simulink model "WindFarm_2023_BaseModel_v2"  (R2019a)
settings: Solver=ode1  StartTime=0.0  StopTime=2  FixedStep=Ts_Power  RelTol=1e-3
PostLoadFcn:
  | %% Init for wind PnO models - global system parameters
  | OVERRIDE_SSN_MEMORY_LIMIT=1;
  | Ts=50e-6;
  | % Ts=50e-10;
  | Ts_Power=Ts;
  | Ts_Control=2*Ts;
  | freq = 50;
  | Fnom=freq;
  | Vac=400e3;
InitFcn:
  | %% Init for wind PnO models - global system parameters
  | OVERRIDE_SSN_MEMORY_LIMIT=1;
  | Ts=50e-6;
  | % Ts=50e-10;
  | Ts_Power=Ts;
  | Ts_Control=2*Ts;
  | freq = 50;
  | Fnom=freq;
  | Vac=400e3;
undefined symbols (not defined in the file or in its folder): Bessel, Butterworth, Complex, D11, Delta, den, DiscIntNeverNeededParam, dx, find_system, gcbh, Iabc, No, num, out_Buses, out_WindFarms, sps_rtmsupport, Vabc, WindFarm_Selection_1, yes
libraries: powerlib x1158, simulink x592, powerlib_meascontrol x592, eeSinusoidalMeasurement x212, simulink_extras x104, elements x52, eePowerMeasurement x50, spsVIMeasurementModel x45
(part 82 of 86)

== system WindFarm_2023_BaseModel_v2/SM_WT1/Wind Type IV Detailed v2.1 - 2/Control/Measurement and Transformation/Discrete 3-phase PLL-Driven Positive-Sequence Active & Reactive Power/Discrete 3-phase PLL-Driven Positive-Sequence Fundamental Value2/Discrete Variable Frequency Mean value1/Correction subsystem ==
  N : Inport
  F : Inport  Port=2
  In : Inport  Port=3
  Gain1 : Gain  Gain=0.5  SaturateOnIntegerOverflow=on  OutDataTypeStr=Inherit: Same as input  ParamDataTypeStr=Inherit: Same as input
  Product2 : Product  Inputs=*/  SaturateOnIntegerOverflow=on  InputSameDT=on  OutDataTypeStr=Inherit: Same as first input
  Product4 : Product  Inputs=**  SaturateOnIntegerOverflow=on  InputSameDT=on  OutDataTypeStr=Inherit: Same as first input
  Product5 : Product  Inputs=**  SaturateOnIntegerOverflow=on  InputSameDT=on  OutDataTypeStr=Inherit: Same as first input
  Sum1 : Sum  Inputs=+-  SaturateOnIntegerOverflow=on  InputSameDT=on  OutDataTypeStr=Inherit: Same as first input
  Sum4 : Sum  SaturateOnIntegerOverflow=on  InputSameDT=on  OutDataTypeStr=Inherit: Same as first input
  Sum5 : Sum  Inputs=+-  SaturateOnIntegerOverflow=on  InputSameDT=on  OutDataTypeStr=Inherit: Same as first input
  Unit Delay : UnitDelay  SampleTime=Ts  HasFrameUpgradeWarning=on
  Out : Outport  VectorParamsAs1DForOutWhenUnconnected=on
  wires:
  Product4/1 -> Out/1
  Sum4/1 -> Product4/2
  Gain1/1 -> Sum4/1
  Product5/1 -> Gain1/1
  Sum1/1 -> Product5/2
  In/1 -> Sum4/2, Unit Delay/1, Sum1/1
  Product2/1 -> Product4/1
  Sum5/1 -> Product5/1, Product2/1
  F/1 -> Sum5/2
  N/1 -> Product2/2, Sum5/1
  Unit Delay/1 -> Sum1/2

== system WindFarm_2023_BaseModel_v2/SM_WT1/Wind Type IV Detailed v2.1 - 2/Control/Measurement and Transformation/Discrete 3-phase PLL-Driven Positive-Sequence Active & Reactive Power/Discrete 3-phase PLL-Driven Positive-Sequence Fundamental Value2/Discrete Variable Frequency Mean value1/Discrete Variable Transport Delay ==
  In : Inport
  D : Inport  Port=2
  "S-Function " : S-Function  FunctionName=discreteVariableTransportDelay  Parameters=MaxDelay,Ts,InitialValue  SFunctionDeploymentMode=off  EnableBusSupport=off
  Out : Outport  VectorParamsAs1DForOutWhenUnconnected=on
  wires:
  D/1 -> "S-Function "/2
  In/1 -> "S-Function "/1
  "S-Function "/1 -> Out/1

== system WindFarm_2023_BaseModel_v2/SM_WT1/Wind Type IV Detailed v2.1 - 2/Control/Measurement and Transformation/Discrete 3-phase PLL-Driven Positive-Sequence Active & Reactive Power/Discrete 3-phase PLL-Driven Positive-Sequence Fundamental Value2/Discrete Variable Frequency Mean value2/Correction subsystem ==
  N : Inport
  F : Inport  Port=2
  In : Inport  Port=3
  Gain1 : Gain  Gain=0.5  SaturateOnIntegerOverflow=on  OutDataTypeStr=Inherit: Same as input  ParamDataTypeStr=Inherit: Same as input
  Product2 : Product  Inputs=*/  SaturateOnIntegerOverflow=on  InputSameDT=on  OutDataTypeStr=Inherit: Same as first input
  Product4 : Product  Inputs=**  SaturateOnIntegerOverflow=on  InputSameDT=on  OutDataTypeStr=Inherit: Same as first input
  Product5 : Product  Inputs=**  SaturateOnIntegerOverflow=on  InputSameDT=on  OutDataTypeStr=Inherit: Same as first input
  Sum1 : Sum  Inputs=+-  SaturateOnIntegerOverflow=on  InputSameDT=on  OutDataTypeStr=Inherit: Same as first input
  Sum4 : Sum  SaturateOnIntegerOverflow=on  InputSameDT=on  OutDataTypeStr=Inherit: Same as first input
  Sum5 : Sum  Inputs=+-  SaturateOnIntegerOverflow=on  InputSameDT=on  OutDataTypeStr=Inherit: Same as first input
  Unit Delay : UnitDelay  SampleTime=Ts  HasFrameUpgradeWarning=on
  Out : Outport  VectorParamsAs1DForOutWhenUnconnected=on
  wires:
  Unit Delay/1 -> Sum1/2
  N/1 -> Sum5/1, Product2/2
  F/1 -> Sum5/2
  Sum5/1 -> Product2/1, Product5/1
  Product2/1 -> Product4/1
  In/1 -> Sum1/1, Unit Delay/1, Sum4/2
  Sum1/1 -> Product5/2
  Product5/1 -> Gain1/1
  Gain1/1 -> Sum4/1
  Sum4/1 -> Product4/2
  Product4/1 -> Out/1

== system WindFarm_2023_BaseModel_v2/SM_WT1/Wind Type IV Detailed v2.1 - 2/Control/Measurement and Transformation/Discrete 3-phase PLL-Driven Positive-Sequence Active & Reactive Power/Discrete 3-phase PLL-Driven Positive-Sequence Fundamental Value2/Discrete Variable Frequency Mean value2/Discrete Variable Transport Delay ==
  In : Inport
  D : Inport  Port=2
  "S-Function " : S-Function  FunctionName=discreteVariableTransportDelay  Parameters=MaxDelay,Ts,InitialValue  SFunctionDeploymentMode=off  EnableBusSupport=off
  Out : Outport  VectorParamsAs1DForOutWhenUnconnected=on
  wires:
  "S-Function "/1 -> Out/1
  In/1 -> "S-Function "/1
  D/1 -> "S-Function "/2

== system WindFarm_2023_BaseModel_v2/SM_WT1/Wind Type IV Detailed v2.1 - 20/Control/Measurement and Transformation/Discrete 3-phase PLL-Driven Positive-Sequence Active & Reactive Power/Discrete 3-phase PLL-Driven Positive-Sequence Fundamental Value/Discrete Variable Frequency Mean value1/Correction subsystem ==
  N : Inport
  F : Inport  Port=2
  In : Inport  Port=3
  Gain1 : Gain  Gain=0.5  SaturateOnIntegerOverflow=on  OutDataTypeStr=Inherit: Same as input  ParamDataTypeStr=Inherit: Same as input
  Product2 : Product  Inputs=*/  SaturateOnIntegerOverflow=on  InputSameDT=on  OutDataTypeStr=Inherit: Same as first input
  Product4 : Product  Inputs=**  SaturateOnIntegerOverflow=on  InputSameDT=on  OutDataTypeStr=Inherit: Same as first input
  Product5 : Product  Inputs=**  SaturateOnIntegerOverflow=on  InputSameDT=on  OutDataTypeStr=Inherit: Same as first input
  Sum1 : Sum  Inputs=+-  SaturateOnIntegerOverflow=on  InputSameDT=on  OutDataTypeStr=Inherit: Same as first input
  Sum4 : Sum  SaturateOnIntegerOverflow=on  InputSameDT=on  OutDataTypeStr=Inherit: Same as first input
  Sum5 : Sum  Inputs=+-  SaturateOnIntegerOverflow=on  InputSameDT=on  OutDataTypeStr=Inherit: Same as first input
  Unit Delay : UnitDelay  SampleTime=Ts  HasFrameUpgradeWarning=on
  Out : Outport  VectorParamsAs1DForOutWhenUnconnected=on
  wires:
  Product4/1 -> Out/1
  Sum4/1 -> Product4/2
  Gain1/1 -> Sum4/1
  Product5/1 -> Gain1/1
  Sum1/1 -> Product5/2
  In/1 -> Sum4/2, Unit Delay/1, Sum1/1
  Product2/1 -> Product4/1
  Sum5/1 -> Product5/1, Product2/1
  F/1 -> Sum5/2
  N/1 -> Product2/2, Sum5/1
  Unit Delay/1 -> Sum1/2

== system WindFarm_2023_BaseModel_v2/SM_WT1/Wind Type IV Detailed v2.1 - 20/Control/Measurement and Transformation/Discrete 3-phase PLL-Driven Positive-Sequence Active & Reactive Power/Discrete 3-phase PLL-Driven Positive-Sequence Fundamental Value/Discrete Variable Frequency Mean value1/Discrete Variable Transport Delay ==
  In : Inport
  D : Inport  Port=2
  "S-Function " : S-Function  FunctionName=discreteVariableTransportDelay  Parameters=MaxDelay,Ts,InitialValue  SFunctionDeploymentMode=off  EnableBusSupport=off
  Out : Outport  VectorParamsAs1DForOutWhenUnconnected=on
  wires:
  D/1 -> "S-Function "/2
  In/1 -> "S-Function "/1
  "S-Function "/1 -> Out/1

== system WindFarm_2023_BaseModel_v2/SM_WT1/Wind Type IV Detailed v2.1 - 20/Control/Measurement and Transformation/Discrete 3-phase PLL-Driven Positive-Sequence Active & Reactive Power/Discrete 3-phase PLL-Driven Positive-Sequence Fundamental Value/Discrete Variable Frequency Mean value2/Correction subsystem ==
  N : Inport
  F : Inport  Port=2
  In : Inport  Port=3
  Gain1 : Gain  Gain=0.5  SaturateOnIntegerOverflow=on  OutDataTypeStr=Inherit: Same as input  ParamDataTypeStr=Inherit: Same as input
  Product2 : Product  Inputs=*/  SaturateOnIntegerOverflow=on  InputSameDT=on  OutDataTypeStr=Inherit: Same as first input
  Product4 : Product  Inputs=**  SaturateOnIntegerOverflow=on  InputSameDT=on  OutDataTypeStr=Inherit: Same as first input
  Product5 : Product  Inputs=**  SaturateOnIntegerOverflow=on  InputSameDT=on  OutDataTypeStr=Inherit: Same as first input
  Sum1 : Sum  Inputs=+-  SaturateOnIntegerOverflow=on  InputSameDT=on  OutDataTypeStr=Inherit: Same as first input
  Sum4 : Sum  SaturateOnIntegerOverflow=on  InputSameDT=on  OutDataTypeStr=Inherit: Same as first input
  Sum5 : Sum  Inputs=+-  SaturateOnIntegerOverflow=on  InputSameDT=on  OutDataTypeStr=Inherit: Same as first input
  Unit Delay : UnitDelay  SampleTime=Ts  HasFrameUpgradeWarning=on
  Out : Outport  VectorParamsAs1DForOutWhenUnconnected=on
  wires:
  Unit Delay/1 -> Sum1/2
  N/1 -> Sum5/1, Product2/2
  F/1 -> Sum5/2
  Sum5/1 -> Product2/1, Product5/1
  Product2/1 -> Product4/1
  In/1 -> Sum1/1, Unit Delay/1, Sum4/2
  Sum1/1 -> Product5/2
  Product5/1 -> Gain1/1
  Gain1/1 -> Sum4/1
  Sum4/1 -> Product4/2
  Product4/1 -> Out/1

== system WindFarm_2023_BaseModel_v2/SM_WT1/Wind Type IV Detailed v2.1 - 20/Control/Measurement and Transformation/Discrete 3-phase PLL-Driven Positive-Sequence Active & Reactive Power/Discrete 3-phase PLL-Driven Positive-Sequence Fundamental Value/Discrete Variable Frequency Mean value2/Discrete Variable Transport Delay ==
  In : Inport
  D : Inport  Port=2
  "S-Function " : S-Function  FunctionName=discreteVariableTransportDelay  Parameters=MaxDelay,Ts,InitialValue  SFunctionDeploymentMode=off  EnableBusSupport=off
  Out : Outport  VectorParamsAs1DForOutWhenUnconnected=on
  wires:
  "S-Function "/1 -> Out/1
  In/1 -> "S-Function "/1
  D/1 -> "S-Function "/2

== system WindFarm_2023_BaseModel_v2/SM_WT1/Wind Type IV Detailed v2.1 - 20/Control/Measurement and Transformation/Discrete 3-phase PLL-Driven Positive-Sequence Active & Reactive Power/Discrete 3-phase PLL-Driven Positive-Sequence Fundamental Value2/Discrete Variable Frequency Mean value1/Correction subsystem ==
  N : Inport
  F : Inport  Port=2
  In : Inport  Port=3
  Gain1 : Gain  Gain=0.5  SaturateOnIntegerOverflow=on  OutDataTypeStr=Inherit: Same as input  ParamDataTypeStr=Inherit: Same as input
  Product2 : Product  Inputs=*/  SaturateOnIntegerOverflow=on  InputSameDT=on  OutDataTypeStr=Inherit: Same as first input
  Product4 : Product  Inputs=**  SaturateOnIntegerOverflow=on  InputSameDT=on  OutDataTypeStr=Inherit: Same as first input
  Product5 : Product  Inputs=**  SaturateOnIntegerOverflow=on  InputSameDT=on  OutDataTypeStr=Inherit: Same as first input
  Sum1 : Sum  Inputs=+-  SaturateOnIntegerOverflow=on  InputSameDT=on  OutDataTypeStr=Inherit: Same as first input
  Sum4 : Sum  SaturateOnIntegerOverflow=on  InputSameDT=on  OutDataTypeStr=Inherit: Same as first input
  Sum5 : Sum  Inputs=+-  SaturateOnIntegerOverflow=on  InputSameDT=on  OutDataTypeStr=Inherit: Same as first input
  Unit Delay : UnitDelay  SampleTime=Ts  HasFrameUpgradeWarning=on
  Out : Outport  VectorParamsAs1DForOutWhenUnconnected=on
  wires:
  Unit Delay/1 -> Sum1/2
  N/1 -> Sum5/1, Product2/2
  F/1 -> Sum5/2
  Sum5/1 -> Product2/1, Product5/1
  Product2/1 -> Product4/1
  In/1 -> Sum1/1, Unit Delay/1, Sum4/2
  Sum1/1 -> Product5/2
  Product5/1 -> Gain1/1
  Gain1/1 -> Sum4/1
  Sum4/1 -> Product4/2
  Product4/1 -> Out/1

== system WindFarm_2023_BaseModel_v2/SM_WT1/Wind Type IV Detailed v2.1 - 20/Control/Measurement and Transformation/Discrete 3-phase PLL-Driven Positive-Sequence Active & Reactive Power/Discrete 3-phase PLL-Driven Positive-Sequence Fundamental Value2/Discrete Variable Frequency Mean value1/Discrete Variable Transport Delay ==
  In : Inport
  D : Inport  Port=2
  "S-Function " : S-Function  FunctionName=discreteVariableTransportDelay  Parameters=MaxDelay,Ts,InitialValue  SFunctionDeploymentMode=off  EnableBusSupport=off
  Out : Outport  VectorParamsAs1DForOutWhenUnconnected=on
  wires:
  "S-Function "/1 -> Out/1
  In/1 -> "S-Function "/1
  D/1 -> "S-Function "/2

== system WindFarm_2023_BaseModel_v2/SM_WT1/Wind Type IV Detailed v2.1 - 20/Control/Measurement and Transformation/Discrete 3-phase PLL-Driven Positive-Sequence Active & Reactive Power/Discrete 3-phase PLL-Driven Positive-Sequence Fundamental Value2/Discrete Variable Frequency Mean value2/Correction subsystem ==
  N : Inport
  F : Inport  Port=2
  In : Inport  Port=3
  Gain1 : Gain  Gain=0.5  SaturateOnIntegerOverflow=on  OutDataTypeStr=Inherit: Same as input  ParamDataTypeStr=Inherit: Same as input
  Product2 : Product  Inputs=*/  SaturateOnIntegerOverflow=on  InputSameDT=on  OutDataTypeStr=Inherit: Same as first input
  Product4 : Product  Inputs=**  SaturateOnIntegerOverflow=on  InputSameDT=on  OutDataTypeStr=Inherit: Same as first input
  Product5 : Product  Inputs=**  SaturateOnIntegerOverflow=on  InputSameDT=on  OutDataTypeStr=Inherit: Same as first input
  Sum1 : Sum  Inputs=+-  SaturateOnIntegerOverflow=on  InputSameDT=on  OutDataTypeStr=Inherit: Same as first input
  Sum4 : Sum  SaturateOnIntegerOverflow=on  InputSameDT=on  OutDataTypeStr=Inherit: Same as first input
  Sum5 : Sum  Inputs=+-  SaturateOnIntegerOverflow=on  InputSameDT=on  OutDataTypeStr=Inherit: Same as first input
  Unit Delay : UnitDelay  SampleTime=Ts  HasFrameUpgradeWarning=on
  Out : Outport  VectorParamsAs1DForOutWhenUnconnected=on
  wires:
  Product4/1 -> Out/1
  Sum4/1 -> Product4/2
  Gain1/1 -> Sum4/1
  Product5/1 -> Gain1/1
  Sum1/1 -> Product5/2
  In/1 -> Sum4/2, Unit Delay/1, Sum1/1
  Product2/1 -> Product4/1
  Sum5/1 -> Product5/1, Product2/1
  F/1 -> Sum5/2
  N/1 -> Product2/2, Sum5/1
  Unit Delay/1 -> Sum1/2

== system WindFarm_2023_BaseModel_v2/SM_WT1/Wind Type IV Detailed v2.1 - 20/Control/Measurement and Transformation/Discrete 3-phase PLL-Driven Positive-Sequence Active & Reactive Power/Discrete 3-phase PLL-Driven Positive-Sequence Fundamental Value2/Discrete Variable Frequency Mean value2/Discrete Variable Transport Delay ==
  In : Inport
  D : Inport  Port=2
  "S-Function " : S-Function  FunctionName=discreteVariableTransportDelay  Parameters=MaxDelay,Ts,InitialValue  SFunctionDeploymentMode=off  EnableBusSupport=off
  Out : Outport  VectorParamsAs1DForOutWhenUnconnected=on
  wires:
  D/1 -> "S-Function "/2
  In/1 -> "S-Function "/1
  "S-Function "/1 -> Out/1

== system WindFarm_2023_BaseModel_v2/SM_WT1/Wind Type IV Detailed v2.1 - 21/Control/Measurement and Transformation/Discrete 3-phase PLL-Driven Positive-Sequence Active & Reactive Power/Discrete 3-phase PLL-Driven Positive-Sequence Fundamental Value/Discrete Variable Frequency Mean value1/Correction subsystem ==
  N : Inport
  F : Inport  Port=2
  In : Inport  Port=3
  Gain1 : Gain  Gain=0.5  SaturateOnIntegerOverflow=on  OutDataTypeStr=Inherit: Same as input  ParamDataTypeStr=Inherit: Same as input
  Product2 : Product  Inputs=*/  SaturateOnIntegerOverflow=on  InputSameDT=on  OutDataTypeStr=Inherit: Same as first input
  Product4 : Product  Inputs=**  SaturateOnIntegerOverflow=on  InputSameDT=on  OutDataTypeStr=Inherit: Same as first input
  Product5 : Product  Inputs=**  SaturateOnIntegerOverflow=on  InputSameDT=on  OutDataTypeStr=Inherit: Same as first input
  Sum1 : Sum  Inputs=+-  SaturateOnIntegerOverflow=on  InputSameDT=on  OutDataTypeStr=Inherit: Same as first input
  Sum4 : Sum  SaturateOnIntegerOverflow=on  InputSameDT=on  OutDataTypeStr=Inherit: Same as first input
  Sum5 : Sum  Inputs=+-  SaturateOnIntegerOverflow=on  InputSameDT=on  OutDataTypeStr=Inherit: Same as first input
  Unit Delay : UnitDelay  SampleTime=Ts  HasFrameUpgradeWarning=on
  Out : Outport  VectorParamsAs1DForOutWhenUnconnected=on
  wires:
  Product4/1 -> Out/1
  Sum4/1 -> Product4/2
  Gain1/1 -> Sum4/1
  Product5/1 -> Gain1/1
  Sum1/1 -> Product5/2
  In/1 -> Sum4/2, Unit Delay/1, Sum1/1
  Product2/1 -> Product4/1
  Sum5/1 -> Product5/1, Product2/1
  F/1 -> Sum5/2
  N/1 -> Product2/2, Sum5/1
  Unit Delay/1 -> Sum1/2

== system WindFarm_2023_BaseModel_v2/SM_WT1/Wind Type IV Detailed v2.1 - 21/Control/Measurement and Transformation/Discrete 3-phase PLL-Driven Positive-Sequence Active & Reactive Power/Discrete 3-phase PLL-Driven Positive-Sequence Fundamental Value/Discrete Variable Frequency Mean value1/Discrete Variable Transport Delay ==
  In : Inport
  D : Inport  Port=2
  "S-Function " : S-Function  FunctionName=discreteVariableTransportDelay  Parameters=MaxDelay,Ts,InitialValue  SFunctionDeploymentMode=off  EnableBusSupport=off
  Out : Outport  VectorParamsAs1DForOutWhenUnconnected=on
  wires:
  D/1 -> "S-Function "/2
  In/1 -> "S-Function "/1
  "S-Function "/1 -> Out/1

== system WindFarm_2023_BaseModel_v2/SM_WT1/Wind Type IV Detailed v2.1 - 21/Control/Measurement and Transformation/Discrete 3-phase PLL-Driven Positive-Sequence Active & Reactive Power/Discrete 3-phase PLL-Driven Positive-Sequence Fundamental Value/Discrete Variable Frequency Mean value2/Correction subsystem ==
  N : Inport
  F : Inport  Port=2
  In : Inport  Port=3
  Gain1 : Gain  Gain=0.5  SaturateOnIntegerOverflow=on  OutDataTypeStr=Inherit: Same as input  ParamDataTypeStr=Inherit: Same as input
  Product2 : Product  Inputs=*/  SaturateOnIntegerOverflow=on  InputSameDT=on  OutDataTypeStr=Inherit: Same as first input
  Product4 : Product  Inputs=**  SaturateOnIntegerOverflow=on  InputSameDT=on  OutDataTypeStr=Inherit: Same as first input
  Product5 : Product  Inputs=**  SaturateOnIntegerOverflow=on  InputSameDT=on  OutDataTypeStr=Inherit: Same as first input
  Sum1 : Sum  Inputs=+-  SaturateOnIntegerOverflow=on  InputSameDT=on  OutDataTypeStr=Inherit: Same as first input
  Sum4 : Sum  SaturateOnIntegerOverflow=on  InputSameDT=on  OutDataTypeStr=Inherit: Same as first input
  Sum5 : Sum  Inputs=+-  SaturateOnIntegerOverflow=on  InputSameDT=on  OutDataTypeStr=Inherit: Same as first input
  Unit Delay : UnitDelay  SampleTime=Ts  HasFrameUpgradeWarning=on
  Out : Outport  VectorParamsAs1DForOutWhenUnconnected=on
  wires:
  Unit Delay/1 -> Sum1/2
  N/1 -> Sum5/1, Product2/2
  F/1 -> Sum5/2
  Sum5/1 -> Product2/1, Product5/1
  Product2/1 -> Product4/1
  In/1 -> Sum1/1, Unit Delay/1, Sum4/2
  Sum1/1 -> Product5/2
  Product5/1 -> Gain1/1
  Gain1/1 -> Sum4/1
  Sum4/1 -> Product4/2
  Product4/1 -> Out/1

== system WindFarm_2023_BaseModel_v2/SM_WT1/Wind Type IV Detailed v2.1 - 21/Control/Measurement and Transformation/Discrete 3-phase PLL-Driven Positive-Sequence Active & Reactive Power/Discrete 3-phase PLL-Driven Positive-Sequence Fundamental Value/Discrete Variable Frequency Mean value2/Discrete Variable Transport Delay ==
  In : Inport
  D : Inport  Port=2
  "S-Function " : S-Function  FunctionName=discreteVariableTransportDelay  Parameters=MaxDelay,Ts,InitialValue  SFunctionDeploymentMode=off  EnableBusSupport=off
  Out : Outport  VectorParamsAs1DForOutWhenUnconnected=on
  wires:
  "S-Function "/1 -> Out/1
  In/1 -> "S-Function "/1
  D/1 -> "S-Function "/2

== system WindFarm_2023_BaseModel_v2/SM_WT1/Wind Type IV Detailed v2.1 - 21/Control/Measurement and Transformation/Discrete 3-phase PLL-Driven Positive-Sequence Active & Reactive Power/Discrete 3-phase PLL-Driven Positive-Sequence Fundamental Value2/Discrete Variable Frequency Mean value1/Correction subsystem ==
  N : Inport
  F : Inport  Port=2
  In : Inport  Port=3
  Gain1 : Gain  Gain=0.5  SaturateOnIntegerOverflow=on  OutDataTypeStr=Inherit: Same as input  ParamDataTypeStr=Inherit: Same as input
  Product2 : Product  Inputs=*/  SaturateOnIntegerOverflow=on  InputSameDT=on  OutDataTypeStr=Inherit: Same as first input
  Product4 : Product  Inputs=**  SaturateOnIntegerOverflow=on  InputSameDT=on  OutDataTypeStr=Inherit: Same as first input
  Product5 : Product  Inputs=**  SaturateOnIntegerOverflow=on  InputSameDT=on  OutDataTypeStr=Inherit: Same as first input
  Sum1 : Sum  Inputs=+-  SaturateOnIntegerOverflow=on  InputSameDT=on  OutDataTypeStr=Inherit: Same as first input
  Sum4 : Sum  SaturateOnIntegerOverflow=on  InputSameDT=on  OutDataTypeStr=Inherit: Same as first input
  Sum5 : Sum  Inputs=+-  SaturateOnIntegerOverflow=on  InputSameDT=on  OutDataTypeStr=Inherit: Same as first input
  Unit Delay : UnitDelay  SampleTime=Ts  HasFrameUpgradeWarning=on
  Out : Outport  VectorParamsAs1DForOutWhenUnconnected=on
  wires:
  Unit Delay/1 -> Sum1/2
  N/1 -> Sum5/1, Product2/2
  F/1 -> Sum5/2
  Sum5/1 -> Product2/1, Product5/1
  Product2/1 -> Product4/1
  In/1 -> Sum1/1, Unit Delay/1, Sum4/2
  Sum1/1 -> Product5/2
  Product5/1 -> Gain1/1
  Gain1/1 -> Sum4/1
  Sum4/1 -> Product4/2
  Product4/1 -> Out/1

== system WindFarm_2023_BaseModel_v2/SM_WT1/Wind Type IV Detailed v2.1 - 21/Control/Measurement and Transformation/Discrete 3-phase PLL-Driven Positive-Sequence Active & Reactive Power/Discrete 3-phase PLL-Driven Positive-Sequence Fundamental Value2/Discrete Variable Frequency Mean value1/Discrete Variable Transport Delay ==
  In : Inport
  D : Inport  Port=2
  "S-Function " : S-Function  FunctionName=discreteVariableTransportDelay  Parameters=MaxDelay,Ts,InitialValue  SFunctionDeploymentMode=off  EnableBusSupport=off
  Out : Outport  VectorParamsAs1DForOutWhenUnconnected=on
  wires:
  "S-Function "/1 -> Out/1
  In/1 -> "S-Function "/1
  D/1 -> "S-Function "/2

== system WindFarm_2023_BaseModel_v2/SM_WT1/Wind Type IV Detailed v2.1 - 21/Control/Measurement and Transformation/Discrete 3-phase PLL-Driven Positive-Sequence Active & Reactive Power/Discrete 3-phase PLL-Driven Positive-Sequence Fundamental Value2/Discrete Variable Frequency Mean value2/Correction subsystem ==
  N : Inport
  F : Inport  Port=2
  In : Inport  Port=3
  Gain1 : Gain  Gain=0.5  SaturateOnIntegerOverflow=on  OutDataTypeStr=Inherit: Same as input  ParamDataTypeStr=Inherit: Same as input
  Product2 : Product  Inputs=*/  SaturateOnIntegerOverflow=on  InputSameDT=on  OutDataTypeStr=Inherit: Same as first input
  Product4 : Product  Inputs=**  SaturateOnIntegerOverflow=on  InputSameDT=on  OutDataTypeStr=Inherit: Same as first input
  Product5 : Product  Inputs=**  SaturateOnIntegerOverflow=on  InputSameDT=on  OutDataTypeStr=Inherit: Same as first input
  Sum1 : Sum  Inputs=+-  SaturateOnIntegerOverflow=on  InputSameDT=on  OutDataTypeStr=Inherit: Same as first input
  Sum4 : Sum  SaturateOnIntegerOverflow=on  InputSameDT=on  OutDataTypeStr=Inherit: Same as first input
  Sum5 : Sum  Inputs=+-  SaturateOnIntegerOverflow=on  InputSameDT=on  OutDataTypeStr=Inherit: Same as first input
  Unit Delay : UnitDelay  SampleTime=Ts  HasFrameUpgradeWarning=on
  Out : Outport  VectorParamsAs1DForOutWhenUnconnected=on
  wires:
  Product4/1 -> Out/1
  Sum4/1 -> Product4/2
  Gain1/1 -> Sum4/1
  Product5/1 -> Gain1/1
  Sum1/1 -> Product5/2
  In/1 -> Sum4/2, Unit Delay/1, Sum1/1
  Product2/1 -> Product4/1
  Sum5/1 -> Product5/1, Product2/1
  F/1 -> Sum5/2
  N/1 -> Product2/2, Sum5/1
  Unit Delay/1 -> Sum1/2

== system WindFarm_2023_BaseModel_v2/SM_WT1/Wind Type IV Detailed v2.1 - 21/Control/Measurement and Transformation/Discrete 3-phase PLL-Driven Positive-Sequence Active & Reactive Power/Discrete 3-phase PLL-Driven Positive-Sequence Fundamental Value2/Discrete Variable Frequency Mean value2/Discrete Variable Transport Delay ==
  In : Inport
  D : Inport  Port=2
  "S-Function " : S-Function  FunctionName=discreteVariableTransportDelay  Parameters=MaxDelay,Ts,InitialValue  SFunctionDeploymentMode=off  EnableBusSupport=off
  Out : Outport  VectorParamsAs1DForOutWhenUnconnected=on
  wires:
  D/1 -> "S-Function "/2
  In/1 -> "S-Function "/1
  "S-Function "/1 -> Out/1

== system WindFarm_2023_BaseModel_v2/SM_WT1/Wind Type IV Detailed v2.1 - 22/Control/Measurement and Transformation/Discrete 3-phase PLL-Driven Positive-Sequence Active & Reactive Power/Discrete 3-phase PLL-Driven Positive-Sequence Fundamental Value/Discrete Variable Frequency Mean value1/Correction subsystem ==
  N : Inport
  F : Inport  Port=2
  In : Inport  Port=3
  Gain1 : Gain  Gain=0.5  SaturateOnIntegerOverflow=on  OutDataTypeStr=Inherit: Same as input  ParamDataTypeStr=Inherit: Same as input
  Product2 : Product  Inputs=*/  SaturateOnIntegerOverflow=on  InputSameDT=on  OutDataTypeStr=Inherit: Same as first input
  Product4 : Product  Inputs=**  SaturateOnIntegerOverflow=on  InputSameDT=on  OutDataTypeStr=Inherit: Same as first input
  Product5 : Product  Inputs=**  SaturateOnIntegerOverflow=on  InputSameDT=on  OutDataTypeStr=Inherit: Same as first input
  Sum1 : Sum  Inputs=+-  SaturateOnIntegerOverflow=on  InputSameDT=on  OutDataTypeStr=Inherit: Same as first input
  Sum4 : Sum  SaturateOnIntegerOverflow=on  InputSameDT=on  OutDataTypeStr=Inherit: Same as first input
  Sum5 : Sum  Inputs=+-  SaturateOnIntegerOverflow=on  InputSameDT=on  OutDataTypeStr=Inherit: Same as first input
  Unit Delay : UnitDelay  SampleTime=Ts  HasFrameUpgradeWarning=on
  Out : Outport  VectorParamsAs1DForOutWhenUnconnected=on
  wires:
  Product4/1 -> Out/1
  Sum4/1 -> Product4/2
  Gain1/1 -> Sum4/1
  Product5/1 -> Gain1/1
  Sum1/1 -> Product5/2
  In/1 -> Sum4/2, Unit Delay/1, Sum1/1
  Product2/1 -> Product4/1
  Sum5/1 -> Product5/1, Product2/1
  F/1 -> Sum5/2
  N/1 -> Product2/2, Sum5/1
  Unit Delay/1 -> Sum1/2

== system WindFarm_2023_BaseModel_v2/SM_WT1/Wind Type IV Detailed v2.1 - 22/Control/Measurement and Transformation/Discrete 3-phase PLL-Driven Positive-Sequence Active & Reactive Power/Discrete 3-phase PLL-Driven Positive-Sequence Fundamental Value/Discrete Variable Frequency Mean value1/Discrete Variable Transport Delay ==
  In : Inport
  D : Inport  Port=2
  "S-Function " : S-Function  FunctionName=discreteVariableTransportDelay  Parameters=MaxDelay,Ts,InitialValue  SFunctionDeploymentMode=off  EnableBusSupport=off
  Out : Outport  VectorParamsAs1DForOutWhenUnconnected=on
  wires:
  D/1 -> "S-Function "/2
  In/1 -> "S-Function "/1
  "S-Function "/1 -> Out/1

== system WindFarm_2023_BaseModel_v2/SM_WT1/Wind Type IV Detailed v2.1 - 22/Control/Measurement and Transformation/Discrete 3-phase PLL-Driven Positive-Sequence Active & Reactive Power/Discrete 3-phase PLL-Driven Positive-Sequence Fundamental Value/Discrete Variable Frequency Mean value2/Correction subsystem ==
  N : Inport
  F : Inport  Port=2
  In : Inport  Port=3
  Gain1 : Gain  Gain=0.5  SaturateOnIntegerOverflow=on  OutDataTypeStr=Inherit: Same as input  ParamDataTypeStr=Inherit: Same as input
  Product2 : Product  Inputs=*/  SaturateOnIntegerOverflow=on  InputSameDT=on  OutDataTypeStr=Inherit: Same as first input
  Product4 : Product  Inputs=**  SaturateOnIntegerOverflow=on  InputSameDT=on  OutDataTypeStr=Inherit: Same as first input
  Product5 : Product  Inputs=**  SaturateOnIntegerOverflow=on  InputSameDT=on  OutDataTypeStr=Inherit: Same as first input
  Sum1 : Sum  Inputs=+-  SaturateOnIntegerOverflow=on  InputSameDT=on  OutDataTypeStr=Inherit: Same as first input
  Sum4 : Sum  SaturateOnIntegerOverflow=on  InputSameDT=on  OutDataTypeStr=Inherit: Same as first input
  Sum5 : Sum  Inputs=+-  SaturateOnIntegerOverflow=on  InputSameDT=on  OutDataTypeStr=Inherit: Same as first input
  Unit Delay : UnitDelay  SampleTime=Ts  HasFrameUpgradeWarning=on
  Out : Outport  VectorParamsAs1DForOutWhenUnconnected=on
  wires:
  Unit Delay/1 -> Sum1/2
  N/1 -> Sum5/1, Product2/2
  F/1 -> Sum5/2
  Sum5/1 -> Product2/1, Product5/1
  Product2/1 -> Product4/1
  In/1 -> Sum1/1, Unit Delay/1, Sum4/2
  Sum1/1 -> Product5/2
  Product5/1 -> Gain1/1
  Gain1/1 -> Sum4/1
  Sum4/1 -> Product4/2
  Product4/1 -> Out/1

== system WindFarm_2023_BaseModel_v2/SM_WT1/Wind Type IV Detailed v2.1 - 22/Control/Measurement and Transformation/Discrete 3-phase PLL-Driven Positive-Sequence Active & Reactive Power/Discrete 3-phase PLL-Driven Positive-Sequence Fundamental Value/Discrete Variable Frequency Mean value2/Discrete Variable Transport Delay ==
  In : Inport
  D : Inport  Port=2
  "S-Function " : S-Function  FunctionName=discreteVariableTransportDelay  Parameters=MaxDelay,Ts,InitialValue  SFunctionDeploymentMode=off  EnableBusSupport=off
  Out : Outport  VectorParamsAs1DForOutWhenUnconnected=on
  wires:
  "S-Function "/1 -> Out/1
  In/1 -> "S-Function "/1
  D/1 -> "S-Function "/2

== system WindFarm_2023_BaseModel_v2/SM_WT1/Wind Type IV Detailed v2.1 - 22/Control/Measurement and Transformation/Discrete 3-phase PLL-Driven Positive-Sequence Active & Reactive Power/Discrete 3-phase PLL-Driven Positive-Sequence Fundamental Value2/Discrete Variable Frequency Mean value1/Correction subsystem ==
  N : Inport
  F : Inport  Port=2
  In : Inport  Port=3
  Gain1 : Gain  Gain=0.5  SaturateOnIntegerOverflow=on  OutDataTypeStr=Inherit: Same as input  ParamDataTypeStr=Inherit: Same as input
  Product2 : Product  Inputs=*/  SaturateOnIntegerOverflow=on  InputSameDT=on  OutDataTypeStr=Inherit: Same as first input
  Product4 : Product  Inputs=**  SaturateOnIntegerOverflow=on  InputSameDT=on  OutDataTypeStr=Inherit: Same as first input
  Product5 : Product  Inputs=**  SaturateOnIntegerOverflow=on  InputSameDT=on  OutDataTypeStr=Inherit: Same as first input
  Sum1 : Sum  Inputs=+-  SaturateOnIntegerOverflow=on  InputSameDT=on  OutDataTypeStr=Inherit: Same as first input
  Sum4 : Sum  SaturateOnIntegerOverflow=on  InputSameDT=on  OutDataTypeStr=Inherit: Same as first input
  Sum5 : Sum  Inputs=+-  SaturateOnIntegerOverflow=on  InputSameDT=on  OutDataTypeStr=Inherit: Same as first input
  Unit Delay : UnitDelay  SampleTime=Ts  HasFrameUpgradeWarning=on
  Out : Outport  VectorParamsAs1DForOutWhenUnconnected=on
  wires:
  Unit Delay/1 -> Sum1/2
  N/1 -> Sum5/1, Product2/2
  F/1 -> Sum5/2
  Sum5/1 -> Product2/1, Product5/1
  Product2/1 -> Product4/1
  In/1 -> Sum1/1, Unit Delay/1, Sum4/2
  Sum1/1 -> Product5/2
  Product5/1 -> Gain1/1
  Gain1/1 -> Sum4/1
  Sum4/1 -> Product4/2
  Product4/1 -> Out/1

== system WindFarm_2023_BaseModel_v2/SM_WT1/Wind Type IV Detailed v2.1 - 22/Control/Measurement and Transformation/Discrete 3-phase PLL-Driven Positive-Sequence Active & Reactive Power/Discrete 3-phase PLL-Driven Positive-Sequence Fundamental Value2/Discrete Variable Frequency Mean value1/Discrete Variable Transport Delay ==
  In : Inport
  D : Inport  Port=2
  "S-Function " : S-Function  FunctionName=discreteVariableTransportDelay  Parameters=MaxDelay,Ts,InitialValue  SFunctionDeploymentMode=off  EnableBusSupport=off
  Out : Outport  VectorParamsAs1DForOutWhenUnconnected=on
  wires:
  "S-Function "/1 -> Out/1
  In/1 -> "S-Function "/1
  D/1 -> "S-Function "/2

== system WindFarm_2023_BaseModel_v2/SM_WT1/Wind Type IV Detailed v2.1 - 22/Control/Measurement and Transformation/Discrete 3-phase PLL-Driven Positive-Sequence Active & Reactive Power/Discrete 3-phase PLL-Driven Positive-Sequence Fundamental Value2/Discrete Variable Frequency Mean value2/Correction subsystem ==
  N : Inport
  F : Inport  Port=2
  In : Inport  Port=3
  Gain1 : Gain  Gain=0.5  SaturateOnIntegerOverflow=on  OutDataTypeStr=Inherit: Same as input  ParamDataTypeStr=Inherit: Same as input
  Product2 : Product  Inputs=*/  SaturateOnIntegerOverflow=on  InputSameDT=on  OutDataTypeStr=Inherit: Same as first input
  Product4 : Product  Inputs=**  SaturateOnIntegerOverflow=on  InputSameDT=on  OutDataTypeStr=Inherit: Same as first input
  Product5 : Product  Inputs=**  SaturateOnIntegerOverflow=on  InputSameDT=on  OutDataTypeStr=Inherit: Same as first input
  Sum1 : Sum  Inputs=+-  SaturateOnIntegerOverflow=on  InputSameDT=on  OutDataTypeStr=Inherit: Same as first input
  Sum4 : Sum  SaturateOnIntegerOverflow=on  InputSameDT=on  OutDataTypeStr=Inherit: Same as first input
  Sum5 : Sum  Inputs=+-  SaturateOnIntegerOverflow=on  InputSameDT=on  OutDataTypeStr=Inherit: Same as first input
  Unit Delay : UnitDelay  SampleTime=Ts  HasFrameUpgradeWarning=on
  Out : Outport  VectorParamsAs1DForOutWhenUnconnected=on
  wires:
  Product4/1 -> Out/1
  Sum4/1 -> Product4/2
  Gain1/1 -> Sum4/1
  Product5/1 -> Gain1/1
  Sum1/1 -> Product5/2
  In/1 -> Sum4/2, Unit Delay/1, Sum1/1
  Product2/1 -> Product4/1
  Sum5/1 -> Product5/1, Product2/1
  F/1 -> Sum5/2
  N/1 -> Product2/2, Sum5/1
  Unit Delay/1 -> Sum1/2

== system WindFarm_2023_BaseModel_v2/SM_WT1/Wind Type IV Detailed v2.1 - 22/Control/Measurement and Transformation/Discrete 3-phase PLL-Driven Positive-Sequence Active & Reactive Power/Discrete 3-phase PLL-Driven Positive-Sequence Fundamental Value2/Discrete Variable Frequency Mean value2/Discrete Variable Transport Delay ==
  In : Inport
  D : Inport  Port=2
  "S-Function " : S-Function  FunctionName=discreteVariableTransportDelay  Parameters=MaxDelay,Ts,InitialValue  SFunctionDeploymentMode=off  EnableBusSupport=off
  Out : Outport  VectorParamsAs1DForOutWhenUnconnected=on
  wires:
  D/1 -> "S-Function "/2
  In/1 -> "S-Function "/1
  "S-Function "/1 -> Out/1

== system WindFarm_2023_BaseModel_v2/SM_WT1/Wind Type IV Detailed v2.1 - 23/Control/Measurement and Transformation/Discrete 3-phase PLL-Driven Positive-Sequence Active & Reactive Power/Discrete 3-phase PLL-Driven Positive-Sequence Fundamental Value/Discrete Variable Frequency Mean value1/Correction subsystem ==
  N : Inport
  F : Inport  Port=2
  In : Inport  Port=3
  Gain1 : Gain  Gain=0.5  SaturateOnIntegerOverflow=on  OutDataTypeStr=Inherit: Same as input  ParamDataTypeStr=Inherit: Same as input
  Product2 : Product  Inputs=*/  SaturateOnIntegerOverflow=on  InputSameDT=on  OutDataTypeStr=Inherit: Same as first input
  Product4 : Product  Inputs=**  SaturateOnIntegerOverflow=on  InputSameDT=on  OutDataTypeStr=Inherit: Same as first input
  Product5 : Product  Inputs=**  SaturateOnIntegerOverflow=on  InputSameDT=on  OutDataTypeStr=Inherit: Same as first input
  Sum1 : Sum  Inputs=+-  SaturateOnIntegerOverflow=on  InputSameDT=on  OutDataTypeStr=Inherit: Same as first input
  Sum4 : Sum  SaturateOnIntegerOverflow=on  InputSameDT=on  OutDataTypeStr=Inherit: Same as first input
  Sum5 : Sum  Inputs=+-  SaturateOnIntegerOverflow=on  InputSameDT=on  OutDataTypeStr=Inherit: Same as first input
  Unit Delay : UnitDelay  SampleTime=Ts  HasFrameUpgradeWarning=on
  Out : Outport  VectorParamsAs1DForOutWhenUnconnected=on
  wires:
  Product4/1 -> Out/1
  Sum4/1 -> Product4/2
  Gain1/1 -> Sum4/1
  Product5/1 -> Gain1/1
  Sum1/1 -> Product5/2
  In/1 -> Sum4/2, Unit Delay/1, Sum1/1
  Product2/1 -> Product4/1
  Sum5/1 -> Product5/1, Product2/1
  F/1 -> Sum5/2
  N/1 -> Product2/2, Sum5/1
  Unit Delay/1 -> Sum1/2

== system WindFarm_2023_BaseModel_v2/SM_WT1/Wind Type IV Detailed v2.1 - 23/Control/Measurement and Transformation/Discrete 3-phase PLL-Driven Positive-Sequence Active & Reactive Power/Discrete 3-phase PLL-Driven Positive-Sequence Fundamental Value/Discrete Variable Frequency Mean value1/Discrete Variable Transport Delay ==
  In : Inport
  D : Inport  Port=2
  "S-Function " : S-Function  FunctionName=discreteVariableTransportDelay  Parameters=MaxDelay,Ts,InitialValue  SFunctionDeploymentMode=off  EnableBusSupport=off
  Out : Outport  VectorParamsAs1DForOutWhenUnconnected=on
  wires:
  D/1 -> "S-Function "/2
  In/1 -> "S-Function "/1
  "S-Function "/1 -> Out/1

== system WindFarm_2023_BaseModel_v2/SM_WT1/Wind Type IV Detailed v2.1 - 23/Control/Measurement and Transformation/Discrete 3-phase PLL-Driven Positive-Sequence Active & Reactive Power/Discrete 3-phase PLL-Driven Positive-Sequence Fundamental Value/Discrete Variable Frequency Mean value2/Correction subsystem ==
  N : Inport
  F : Inport  Port=2
  In : Inport  Port=3
  Gain1 : Gain  Gain=0.5  SaturateOnIntegerOverflow=on  OutDataTypeStr=Inherit: Same as input  ParamDataTypeStr=Inherit: Same as input
  Product2 : Product  Inputs=*/  SaturateOnIntegerOverflow=on  InputSameDT=on  OutDataTypeStr=Inherit: Same as first input
  Product4 : Product  Inputs=**  SaturateOnIntegerOverflow=on  InputSameDT=on  OutDataTypeStr=Inherit: Same as first input
  Product5 : Product  Inputs=**  SaturateOnIntegerOverflow=on  InputSameDT=on  OutDataTypeStr=Inherit: Same as first input
  Sum1 : Sum  Inputs=+-  SaturateOnIntegerOverflow=on  InputSameDT=on  OutDataTypeStr=Inherit: Same as first input
  Sum4 : Sum  SaturateOnIntegerOverflow=on  InputSameDT=on  OutDataTypeStr=Inherit: Same as first input
  Sum5 : Sum  Inputs=+-  SaturateOnIntegerOverflow=on  InputSameDT=on  OutDataTypeStr=Inherit: Same as first input
  Unit Delay : UnitDelay  SampleTime=Ts  HasFrameUpgradeWarning=on
  Out : Outport  VectorParamsAs1DForOutWhenUnconnected=on
  wires:
  Unit Delay/1 -> Sum1/2
  N/1 -> Sum5/1, Product2/2
  F/1 -> Sum5/2
  Sum5/1 -> Product2/1, Product5/1
  Product2/1 -> Product4/1
  In/1 -> Sum1/1, Unit Delay/1, Sum4/2
  Sum1/1 -> Product5/2
  Product5/1 -> Gain1/1
  Gain1/1 -> Sum4/1
  Sum4/1 -> Product4/2
  Product4/1 -> Out/1

== system WindFarm_2023_BaseModel_v2/SM_WT1/Wind Type IV Detailed v2.1 - 23/Control/Measurement and Transformation/Discrete 3-phase PLL-Driven Positive-Sequence Active & Reactive Power/Discrete 3-phase PLL-Driven Positive-Sequence Fundamental Value/Discrete Variable Frequency Mean value2/Discrete Variable Transport Delay ==
  In : Inport
  D : Inport  Port=2
  "S-Function " : S-Function  FunctionName=discreteVariableTransportDelay  Parameters=MaxDelay,Ts,InitialValue  SFunctionDeploymentMode=off  EnableBusSupport=off
  Out : Outport  VectorParamsAs1DForOutWhenUnconnected=on
  wires:
  "S-Function "/1 -> Out/1
  In/1 -> "S-Function "/1
  D/1 -> "S-Function "/2

== system WindFarm_2023_BaseModel_v2/SM_WT1/Wind Type IV Detailed v2.1 - 23/Control/Measurement and Transformation/Discrete 3-phase PLL-Driven Positive-Sequence Active & Reactive Power/Discrete 3-phase PLL-Driven Positive-Sequence Fundamental Value2/Discrete Variable Frequency Mean value1/Correction subsystem ==
  N : Inport
  F : Inport  Port=2
  In : Inport  Port=3
  Gain1 : Gain  Gain=0.5  SaturateOnIntegerOverflow=on  OutDataTypeStr=Inherit: Same as input  ParamDataTypeStr=Inherit: Same as input
  Product2 : Product  Inputs=*/  SaturateOnIntegerOverflow=on  InputSameDT=on  OutDataTypeStr=Inherit: Same as first input
  Product4 : Product  Inputs=**  SaturateOnIntegerOverflow=on  InputSameDT=on  OutDataTypeStr=Inherit: Same as first input
  Product5 : Product  Inputs=**  SaturateOnIntegerOverflow=on  InputSameDT=on  OutDataTypeStr=Inherit: Same as first input
  Sum1 : Sum  Inputs=+-  SaturateOnIntegerOverflow=on  InputSameDT=on  OutDataTypeStr=Inherit: Same as first input
  Sum4 : Sum  SaturateOnIntegerOverflow=on  InputSameDT=on  OutDataTypeStr=Inherit: Same as first input
  Sum5 : Sum  Inputs=+-  SaturateOnIntegerOverflow=on  InputSameDT=on  OutDataTypeStr=Inherit: Same as first input
  Unit Delay : UnitDelay  SampleTime=Ts  HasFrameUpgradeWarning=on
  Out : Outport  VectorParamsAs1DForOutWhenUnconnected=on
  wires:
  Unit Delay/1 -> Sum1/2
  N/1 -> Sum5/1, Product2/2
  F/1 -> Sum5/2
  Sum5/1 -> Product2/1, Product5/1
  Product2/1 -> Product4/1
  In/1 -> Sum1/1, Unit Delay/1, Sum4/2
  Sum1/1 -> Product5/2
  Product5/1 -> Gain1/1
  Gain1/1 -> Sum4/1
  Sum4/1 -> Product4/2
  Product4/1 -> Out/1

== system WindFarm_2023_BaseModel_v2/SM_WT1/Wind Type IV Detailed v2.1 - 23/Control/Measurement and Transformation/Discrete 3-phase PLL-Driven Positive-Sequence Active & Reactive Power/Discrete 3-phase PLL-Driven Positive-Sequence Fundamental Value2/Discrete Variable Frequency Mean value1/Discrete Variable Transport Delay ==
  In : Inport
  D : Inport  Port=2
  "S-Function " : S-Function  FunctionName=discreteVariableTransportDelay  Parameters=MaxDelay,Ts,InitialValue  SFunctionDeploymentMode=off  EnableBusSupport=off
  Out : Outport  VectorParamsAs1DForOutWhenUnconnected=on
  wires:
  "S-Function "/1 -> Out/1
  In/1 -> "S-Function "/1
  D/1 -> "S-Function "/2

== system WindFarm_2023_BaseModel_v2/SM_WT1/Wind Type IV Detailed v2.1 - 23/Control/Measurement and Transformation/Discrete 3-phase PLL-Driven Positive-Sequence Active & Reactive Power/Discrete 3-phase PLL-Driven Positive-Sequence Fundamental Value2/Discrete Variable Frequency Mean value2/Correction subsystem ==
  N : Inport
  F : Inport  Port=2
  In : Inport  Port=3
  Gain1 : Gain  Gain=0.5  SaturateOnIntegerOverflow=on  OutDataTypeStr=Inherit: Same as input  ParamDataTypeStr=Inherit: Same as input
  Product2 : Product  Inputs=*/  SaturateOnIntegerOverflow=on  InputSameDT=on  OutDataTypeStr=Inherit: Same as first input
  Product4 : Product  Inputs=**  SaturateOnIntegerOverflow=on  InputSameDT=on  OutDataTypeStr=Inherit: Same as first input
  Product5 : Product  Inputs=**  SaturateOnIntegerOverflow=on  InputSameDT=on  OutDataTypeStr=Inherit: Same as first input
  Sum1 : Sum  Inputs=+-  SaturateOnIntegerOverflow=on  InputSameDT=on  OutDataTypeStr=Inherit: Same as first input
  Sum4 : Sum  SaturateOnIntegerOverflow=on  InputSameDT=on  OutDataTypeStr=Inherit: Same as first input
  Sum5 : Sum  Inputs=+-  SaturateOnIntegerOverflow=on  InputSameDT=on  OutDataTypeStr=Inherit: Same as first input
  Unit Delay : UnitDelay  SampleTime=Ts  HasFrameUpgradeWarning=on
  Out : Outport  VectorParamsAs1DForOutWhenUnconnected=on
  wires:
  Product4/1 -> Out/1
  Sum4/1 -> Product4/2
  Gain1/1 -> Sum4/1
  Product5/1 -> Gain1/1
  Sum1/1 -> Product5/2
  In/1 -> Sum4/2, Unit Delay/1, Sum1/1
  Product2/1 -> Product4/1
  Sum5/1 -> Product5/1, Product2/1
  F/1 -> Sum5/2
  N/1 -> Product2/2, Sum5/1
  Unit Delay/1 -> Sum1/2

== system WindFarm_2023_BaseModel_v2/SM_WT1/Wind Type IV Detailed v2.1 - 23/Control/Measurement and Transformation/Discrete 3-phase PLL-Driven Positive-Sequence Active & Reactive Power/Discrete 3-phase PLL-Driven Positive-Sequence Fundamental Value2/Discrete Variable Frequency Mean value2/Discrete Variable Transport Delay ==
  In : Inport
  D : Inport  Port=2
  "S-Function " : S-Function  FunctionName=discreteVariableTransportDelay  Parameters=MaxDelay,Ts,InitialValue  SFunctionDeploymentMode=off  EnableBusSupport=off
  Out : Outport  VectorParamsAs1DForOutWhenUnconnected=on
  wires:
  D/1 -> "S-Function "/2
  In/1 -> "S-Function "/1
  "S-Function "/1 -> Out/1

== system WindFarm_2023_BaseModel_v2/SM_WT1/Wind Type IV Detailed v2.1 - 24/Control/Measurement and Transformation/Discrete 3-phase PLL-Driven Positive-Sequence Active & Reactive Power/Discrete 3-phase PLL-Driven Positive-Sequence Fundamental Value/Discrete Variable Frequency Mean value1/Correction subsystem ==
  N : Inport
  F : Inport  Port=2
  In : Inport  Port=3
  Gain1 : Gain  Gain=0.5  SaturateOnIntegerOverflow=on  OutDataTypeStr=Inherit: Same as input  ParamDataTypeStr=Inherit: Same as input
  Product2 : Product  Inputs=*/  SaturateOnIntegerOverflow=on  InputSameDT=on  OutDataTypeStr=Inherit: Same as first input
  Product4 : Product  Inputs=**  SaturateOnIntegerOverflow=on  InputSameDT=on  OutDataTypeStr=Inherit: Same as first input
  Product5 : Product  Inputs=**  SaturateOnIntegerOverflow=on  InputSameDT=on  OutDataTypeStr=Inherit: Same as first input
  Sum1 : Sum  Inputs=+-  SaturateOnIntegerOverflow=on  InputSameDT=on  OutDataTypeStr=Inherit: Same as first input
  Sum4 : Sum  SaturateOnIntegerOverflow=on  InputSameDT=on  OutDataTypeStr=Inherit: Same as first input
  Sum5 : Sum  Inputs=+-  SaturateOnIntegerOverflow=on  InputSameDT=on  OutDataTypeStr=Inherit: Same as first input
  Unit Delay : UnitDelay  SampleTime=Ts  HasFrameUpgradeWarning=on
  Out : Outport  VectorParamsAs1DForOutWhenUnconnected=on
  wires:
  Product4/1 -> Out/1
  Sum4/1 -> Product4/2
  Gain1/1 -> Sum4/1
  Product5/1 -> Gain1/1
  Sum1/1 -> Product5/2
  In/1 -> Sum4/2, Unit Delay/1, Sum1/1
  Product2/1 -> Product4/1
  Sum5/1 -> Product5/1, Product2/1
  F/1 -> Sum5/2
  N/1 -> Product2/2, Sum5/1
  Unit Delay/1 -> Sum1/2

== system WindFarm_2023_BaseModel_v2/SM_WT1/Wind Type IV Detailed v2.1 - 24/Control/Measurement and Transformation/Discrete 3-phase PLL-Driven Positive-Sequence Active & Reactive Power/Discrete 3-phase PLL-Driven Positive-Sequence Fundamental Value/Discrete Variable Frequency Mean value1/Discrete Variable Transport Delay ==
  In : Inport
  D : Inport  Port=2
  "S-Function " : S-Function  FunctionName=discreteVariableTransportDelay  Parameters=MaxDelay,Ts,InitialValue  SFunctionDeploymentMode=off  EnableBusSupport=off
  Out : Outport  VectorParamsAs1DForOutWhenUnconnected=on
  wires:
  D/1 -> "S-Function "/2
  In/1 -> "S-Function "/1
  "S-Function "/1 -> Out/1

== system WindFarm_2023_BaseModel_v2/SM_WT1/Wind Type IV Detailed v2.1 - 24/Control/Measurement and Transformation/Discrete 3-phase PLL-Driven Positive-Sequence Active & Reactive Power/Discrete 3-phase PLL-Driven Positive-Sequence Fundamental Value/Discrete Variable Frequency Mean value2/Correction subsystem ==
  N : Inport
  F : Inport  Port=2
  In : Inport  Port=3
  Gain1 : Gain  Gain=0.5  SaturateOnIntegerOverflow=on  OutDataTypeStr=Inherit: Same as input  ParamDataTypeStr=Inherit: Same as input
  Product2 : Product  Inputs=*/  SaturateOnIntegerOverflow=on  InputSameDT=on  OutDataTypeStr=Inherit: Same as first input
  Product4 : Product  Inputs=**  SaturateOnIntegerOverflow=on  InputSameDT=on  OutDataTypeStr=Inherit: Same as first input
  Product5 : Product  Inputs=**  SaturateOnIntegerOverflow=on  InputSameDT=on  OutDataTypeStr=Inherit: Same as first input
  Sum1 : Sum  Inputs=+-  SaturateOnIntegerOverflow=on  InputSameDT=on  OutDataTypeStr=Inherit: Same as first input
  Sum4 : Sum  SaturateOnIntegerOverflow=on  InputSameDT=on  OutDataTypeStr=Inherit: Same as first input
  Sum5 : Sum  Inputs=+-  SaturateOnIntegerOverflow=on  InputSameDT=on  OutDataTypeStr=Inherit: Same as first input
  Unit Delay : UnitDelay  SampleTime=Ts  HasFrameUpgradeWarning=on
  Out : Outport  VectorParamsAs1DForOutWhenUnconnected=on
  wires:
  Unit Delay/1 -> Sum1/2
  N/1 -> Sum5/1, Product2/2
  F/1 -> Sum5/2
  Sum5/1 -> Product2/1, Product5/1
  Product2/1 -> Product4/1
  In/1 -> Sum1/1, Unit Delay/1, Sum4/2
  Sum1/1 -> Product5/2
  Product5/1 -> Gain1/1
  Gain1/1 -> Sum4/1
  Sum4/1 -> Product4/2
  Product4/1 -> Out/1

== system WindFarm_2023_BaseModel_v2/SM_WT1/Wind Type IV Detailed v2.1 - 24/Control/Measurement and Transformation/Discrete 3-phase PLL-Driven Positive-Sequence Active & Reactive Power/Discrete 3-phase PLL-Driven Positive-Sequence Fundamental Value/Discrete Variable Frequency Mean value2/Discrete Variable Transport Delay ==
  In : Inport
  D : Inport  Port=2
  "S-Function " : S-Function  FunctionName=discreteVariableTransportDelay  Parameters=MaxDelay,Ts,InitialValue  SFunctionDeploymentMode=off  EnableBusSupport=off
  Out : Outport  VectorParamsAs1DForOutWhenUnconnected=on
  wires:
  "S-Function "/1 -> Out/1
  In/1 -> "S-Function "/1
  D/1 -> "S-Function "/2

== system WindFarm_2023_BaseModel_v2/SM_WT1/Wind Type IV Detailed v2.1 - 24/Control/Measurement and Transformation/Discrete 3-phase PLL-Driven Positive-Sequence Active & Reactive Power/Discrete 3-phase PLL-Driven Positive-Sequence Fundamental Value2/Discrete Variable Frequency Mean value1/Correction subsystem ==
  N : Inport
  F : Inport  Port=2
  In : Inport  Port=3
  Gain1 : Gain  Gain=0.5  SaturateOnIntegerOverflow=on  OutDataTypeStr=Inherit: Same as input  ParamDataTypeStr=Inherit: Same as input
  Product2 : Product  Inputs=*/  SaturateOnIntegerOverflow=on  InputSameDT=on  OutDataTypeStr=Inherit: Same as first input
  Product4 : Product  Inputs=**  SaturateOnIntegerOverflow=on  InputSameDT=on  OutDataTypeStr=Inherit: Same as first input
  Product5 : Product  Inputs=**  SaturateOnIntegerOverflow=on  InputSameDT=on  OutDataTypeStr=Inherit: Same as first input
  Sum1 : Sum  Inputs=+-  SaturateOnIntegerOverflow=on  InputSameDT=on  OutDataTypeStr=Inherit: Same as first input
  Sum4 : Sum  SaturateOnIntegerOverflow=on  InputSameDT=on  OutDataTypeStr=Inherit: Same as first input
  Sum5 : Sum  Inputs=+-  SaturateOnIntegerOverflow=on  InputSameDT=on  OutDataTypeStr=Inherit: Same as first input
  Unit Delay : UnitDelay  SampleTime=Ts  HasFrameUpgradeWarning=on
  Out : Outport  VectorParamsAs1DForOutWhenUnconnected=on
  wires:
  Unit Delay/1 -> Sum1/2
  N/1 -> Sum5/1, Product2/2
  F/1 -> Sum5/2
  Sum5/1 -> Product2/1, Product5/1
  Product2/1 -> Product4/1
  In/1 -> Sum1/1, Unit Delay/1, Sum4/2
  Sum1/1 -> Product5/2
  Product5/1 -> Gain1/1
  Gain1/1 -> Sum4/1
  Sum4/1 -> Product4/2
  Product4/1 -> Out/1

== system WindFarm_2023_BaseModel_v2/SM_WT1/Wind Type IV Detailed v2.1 - 24/Control/Measurement and Transformation/Discrete 3-phase PLL-Driven Positive-Sequence Active & Reactive Power/Discrete 3-phase PLL-Driven Positive-Sequence Fundamental Value2/Discrete Variable Frequency Mean value1/Discrete Variable Transport Delay ==
  In : Inport
  D : Inport  Port=2
  "S-Function " : S-Function  FunctionName=discreteVariableTransportDelay  Parameters=MaxDelay,Ts,InitialValue  SFunctionDeploymentMode=off  EnableBusSupport=off
  Out : Outport  VectorParamsAs1DForOutWhenUnconnected=on
  wires:
  "S-Function "/1 -> Out/1
  In/1 -> "S-Function "/1
  D/1 -> "S-Function "/2
